simulink model "mecanum_chassis"  (R2024b)
settings: Solver=VariableStepAuto  StartTime=0.0  StopTime=10  RelTol=1e-3
libraries: wheel_chassis x4
settings Model: DataDictionary=mecanum_params.sldd  Creator=Austinchao  LastModifiedBy=Austinchao

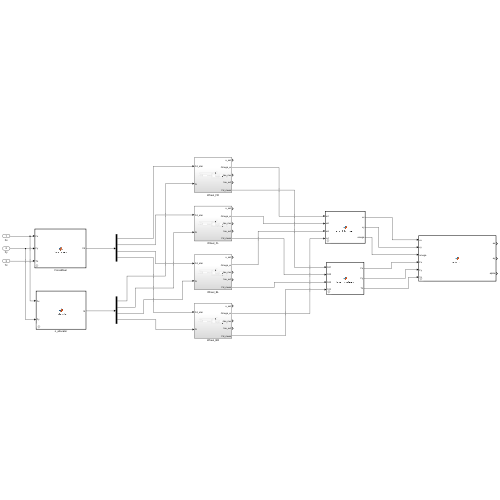
[thumbnail: Simulink's stored preview of the top-level diagram]
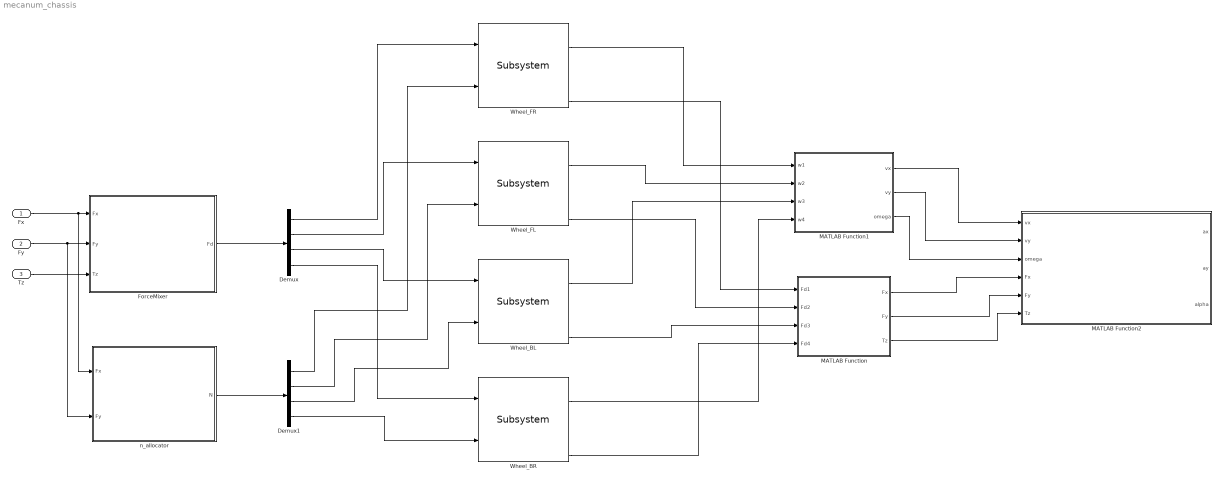
== system mecanum_chassis ==
  Fx : Inport
  Fy : Inport  Port=2
  Tz : Inport  Port=3
  " ForceMixer" : MATLAB Function  TreatAsAtomicUnit=on  mask{a=0, b=0}
      mask prompts: a "Half length (a)"; b "Half width (b)"
  Demux : Demux
  Demux1 : Demux
  MATLAB Function : MATLAB Function  TreatAsAtomicUnit=on  mask{a=0, b=0}
      mask prompts: a "a : left & right (1/2)"; b "b : front & rear (1/2)"
  MATLAB Function1 : MATLAB Function  TreatAsAtomicUnit=on  mask{a=0, b=0, R=0}
      mask prompts: a "a: half length [m]"; b "b: half width [m]"; R "R: wheel radius [m]"
  MATLAB Function2 : MATLAB Function  TreatAsAtomicUnit=on  mask{M=0, Izz=0, bx=0, by=0, bphi=0, useCoriolis=0}
      mask prompts: M "M (Total Mass)"; Izz "Izz (kg.m**2)"
  Wheel_BL : wheel_chassis/Subsystem  SystemSampleTime=-1  VariantActivationTime=update diagram  AllowFlexibleInterface=on  Latency=0  AutoFrameSizeCalculation=off
  Wheel_BR : wheel_chassis/Subsystem  SystemSampleTime=-1  VariantActivationTime=update diagram  AllowFlexibleInterface=on  Latency=0  AutoFrameSizeCalculation=off
  Wheel_FL : wheel_chassis/Subsystem  SystemSampleTime=-1  VariantActivationTime=update diagram  AllowFlexibleInterface=on  Latency=0  AutoFrameSizeCalculation=off
  Wheel_FR : wheel_chassis/Subsystem  SystemSampleTime=-1  VariantActivationTime=update diagram  AllowFlexibleInterface=on  Latency=0  AutoFrameSizeCalculation=off
  n_allocator : MATLAB Function  TreatAsAtomicUnit=on  mask{M=0, g=0, h=0, L=0, W=0}
      mask prompts: M "M : Total mass"; g "g : Gravitational acceleration"; h "h : Center of mass height"; L "L : Wheelbase (front & rear)"; W "W : Track width (right & left)"
  wires:
  Fx/1 -> " ForceMixer"/1(Fx), n_allocator/1(Fx)
  Fy/1 -> " ForceMixer"/2(Fy), n_allocator/2(Fy)
  Tz/1 -> " ForceMixer"/3(Tz)
  " ForceMixer"/1(Fd) -> Demux/1
  Demux/1 -> Wheel_FR/1
  Demux/2 -> Wheel_FL/1
  Demux/3 -> Wheel_BL/1
  Demux/4 -> Wheel_BR/1
  n_allocator/1(N) -> Demux1/1
  Demux1/1 -> Wheel_FR/2
  Demux1/2 -> Wheel_FL/2
  Demux1/3 -> Wheel_BL/2
  Demux1/4 -> Wheel_BR/2
  Wheel_FR/5 -> MATLAB Function/1(Fd1)
  Wheel_FL/5 -> MATLAB Function/2(Fd2)
  Wheel_BL/5 -> MATLAB Function/3(Fd3)
  Wheel_BR/5 -> MATLAB Function/4(Fd4)
  Wheel_FR/2 -> MATLAB Function1/1(w1)
  Wheel_FL/2 -> MATLAB Function1/2(w2)
  Wheel_BL/2 -> MATLAB Function1/3(w3)
  Wheel_BR/2 -> MATLAB Function1/4(w4)
  MATLAB Function1/1(vx) -> MATLAB Function2/1(vx)
  MATLAB Function1/2(vy) -> MATLAB Function2/2(vy)
  MATLAB Function1/3(omega) -> MATLAB Function2/3(omega)
  MATLAB Function/1(Fx) -> MATLAB Function2/4(Fx)
  MATLAB Function/2(Fy) -> MATLAB Function2/5(Fy)
  MATLAB Function/3(Tz) -> MATLAB Function2/6(Tz)

== matlab function mecanum_chassis/ ForceMixer ==
  data: Fx input; Fd output; Fy input; Tz input; a parameter; b parameter
function Fd = force_mixer(Fx, Fy, Tz, a, b)
%#codegen
H = [ -0.5, 0.5, -0.5, 0.5;
       0.5, 0.5,  0.5, 0.5;
      (a+b)/2, -(a+b)/2, -(a+b)/2, (a+b)/2 ];
Fr = [Fx; Fy; Tz];
Fd = (H'/(H*H')) * Fr;
end

== matlab function mecanum_chassis/n_allocator ==
  data: Fx input; N output; Fy input
function N = n_allocator(Fx, Fy)
% Fx: 車體 x 方向的合力 (右正)
% Fy: 車體 y 方向的合力 (前正)

% 計算加速度
ax = Fx / M;
ay = Fy / M;

% 基本參數
N0 = (M*g)/4;
kL = (M*h)/(2*L);
kW = (M*h)/(2*W);

% 四輪分配 [FR, FL, BL, BR]
N = zeros(1,4);
N(1) = N0 - kL*ay - kW*ax;  % FR
N(2) = N0 - kL*ay + kW*ax;  % FL
N(3) = N0 + kL*ay + kW*ax;  % BL
N(4) = N0 + kL*ay - kW*ax;  % BR

% 保護：非負 + 總和守恆
N = max(N,0);
N = N * (M*g / max(sum(N), eps));
end

== matlab function mecanum_chassis/MATLAB Function ==
  data: Fd1 input; Fx output; Fd2 input; Fd3 input; Fd4 input; Fy output; Tz output
function [Fx, Fy, Tz] = force_combiner(Fd1, Fd2, Fd3, Fd4)
% Combine wheel forces into chassis resultant wrench
% Inputs: four wheel measured tangential forces (Fd_meas)
% Params: a = half length (x-direction), b = half width (y-direction)

Fx = 0.5 * (-Fd1 + Fd2 - Fd3 + Fd4);
Fy = 0.5 * ( Fd1 + Fd2 + Fd3 + Fd4);

Tz = 0.5*a*(Fd1 - Fd2 - Fd3 + Fd4) ...
   + 0.5*b*(Fd1 - Fd2 + Fd3 - Fd4);
end

== matlab function mecanum_chassis/MATLAB Function1 ==
  data: w1 input; vx output; w2 input; w3 input; w4 input; vy output; omega output
function [vx, vy, omega] = wheel_kin_body(w1, w2, w3, w4)
% Wheel kinematics → body-frame twist
% w1..w4: wheel angular speeds [rad/s] (1=FR, 2=FL, 3=BL, 4=BR)
% R: wheel radius [m], a: half length [m], b: half width [m]
vx    = (R/4)*(-w1 + w2 - w3 + w4);
vy    = (R/4)*( w1 + w2 + w3 + w4);
omega = (R/(4*(a+b)))*( w1 - w2 - w3 + w4);
end

== matlab function mecanum_chassis/MATLAB Function2 ==
  data: vx input; vy input; omega input; Fx input; ax output; Fy input; Tz input; ay output; alpha output
function [ax, ay, alpha] = body_dyn(vx,vy,omega, Fx,Fy,Tz)
% Body-frame dynamics: forces -> accelerations
% useCoriolis = 0/1 (mask 勾選；先設 0)

if useCoriolis ~= 0
    ax = (Fx - bx*vx)/M + omega*vy;
    ay = (Fy - by*vy)/M - omega*vx;
else
    ax = (Fx - bx*vx)/M;
    ay = (Fy - by*vy)/M;
end
alpha = (Tz - bphi*omega)/Izz;
end
